simulink model "pend_viscous_p1p2_M2019b"  (R2019b)
settings: Solver=FixedStepAuto  StartTime=0.0  StopTime=10  FixedStep=0.01  RelTol=1e-3  EnableMultiTasking=on
values from neighbouring files (symbols this model uses):
  p1 = linspace(0.2,4,n)    [creteFigure3Delipse.m]    (also in viewSavedData.m)
  p2 = linspace(150,250,n)    [creteFigure3Delipse.m]    (also in viewSavedData.m)
  phi0 = linspace(3.5,6.5,n)    [creteFigure3Delipse.m]    (also in viewSavedData.m)
settings Model: Creator=grepl  LastModifiedBy=grepl
settings DataIOCC: LimitDataPoints=on  SaveFormat=Array  SignalLoggingSaveFormat=ModelDataLogs  ReturnWorkspaceOutputs=off
settings OptimizationCC: ExpressionDepthLimit=2147483647  LifeSpan=inf
settings DebuggingCC: UnderspecifiedInitializationDetection=Classic  MergeDetectMultiDrivingBlocksExec=none  FcnCallInpInsideContextMsg=warning  StateNameClashWarn=warning  SFUnexpectedBacktrackingDiag=warning  SFNoUnconditionalDefaultTransitionDiag=warning  SFExecutionAtInitializationDiag=none  ArithmeticOperatorsInVariantConditions=warning
settings HardwareCC: ProdBitPerPointer=32  ProdBitPerSizeT=32  ProdBitPerPtrDiffT=32  ProdLargestAtomicFloat=None  ProdIntDivRoundTo=Undefined  ProdEndianess=Unspecified  ProdWordSize=32  ProdHWDeviceType=32-bit Generic
settings ModelReferenceCC: PropagateSignalLabelsOutOfModel=off
settings SFSimCC: SimUseLocalCustomCode=off  CustomCodeUndefinedFunction=UseInterfaceOnly
settings RTWCC: RTWUseLocalCustomCode=off
settings CodeAppCC: StateflowObjectComments=on
settings GRTTargetCC: TargetLangStandard=C89/C90 (ANSI)  GeneratePreprocessorConditionals=Disable all  CombineOutputUpdateFcns=off  GRTInterface=on
settings ConfigComp: CovMetricSettings=dw  CovHtmlReporting=on  CovSaveCumulativeToWorkspaceVar=on  CovSaveSingleToWorkspaceVar=on  CovExternalEMLEnable=off

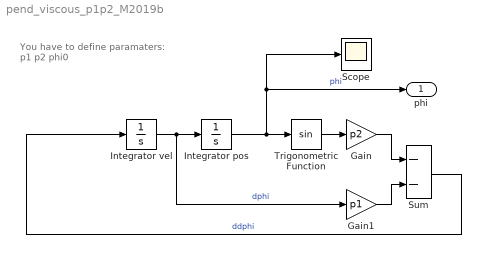
== system pend_viscous_p1p2_M2019b ==
  note: You have to define paramaters:
      | p1
      | p2
      | phi0
  Gain : Gain  Gain=p2
  Gain1 : Gain  Gain=p1
  Integrator pos : Integrator  InitialCondition=phi0
  Integrator vel : Integrator
  Scope : Scope
  Sum : Sum  Inputs=--
  Trigonometric Function : Trigonometry
  phi : Outport
  wires:
  Integrator vel/1 -> Integrator pos/1, Gain1/1  "dphi"
  Sum/1 -> Integrator vel/1  "ddphi"
  Integrator pos/1 -> Trigonometric Function/1, Scope/1, phi/1  "phi"
  Trigonometric Function/1 -> Gain/1
  Gain/1 -> Sum/1
  Gain1/1 -> Sum/2
